simulink model "OuterLoop"  (R2023b)
settings: Solver=VariableStepAuto  StartTime=0.0  StopTime=10.0  RelTol=1e-3
model workspace (MAT data in the model file):
  TorqueSat = 0.0675
values from neighbouring files (symbols this model uses):
  Jb = Js    (= 0.05116)    [Attitude_OuterLoop.m]    (also in SystemVariables.m)
  K = place(A,B,p)    [Attitude_OuterLoop.m]    (also in BLDC_measures.m = 11200)
  Kt = Ke    (= 0.0675)    [Attitude_OuterLoop.m]    (also in BLDC_measures.m; SystemVariables.m)
libraries: simulink_extras x2
settings Model: Creator=Jorge CM  LastModifiedBy=Jorge CM

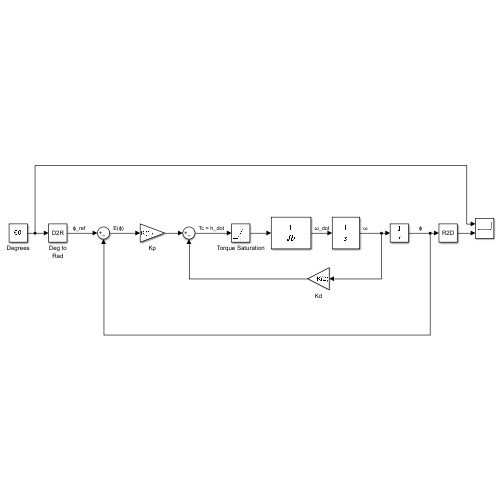
[thumbnail: Simulink's stored preview of the top-level diagram]
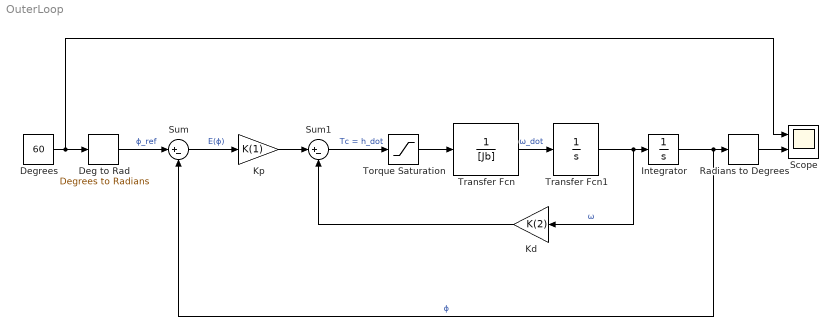
== system OuterLoop ==
  Deg to Rad : simulink_extras/Transformations/Degrees to Radians
  Degrees : Constant  Value=60
  Integrator : Integrator
  Kd : Gain  Gain=K(2)
  Kp : Gain  Gain=K(1)
  Radians to Degrees : simulink_extras/Transformations/Radians to Degrees
  Scope : Scope  NumInputPorts=2
  Sum : Sum  Inputs=|+-
  Sum1 : Sum  Inputs=|+-
  Torque Saturation : Saturate  UpperLimit=Kt  LowerLimit=-Kt
  Transfer Fcn : TransferFcn  Denominator=[Jb]
  Transfer Fcn1 : TransferFcn  Denominator=[1 0]
  wires:
  Degrees/1 -> Scope/1, Deg to Rad/1
  Deg to Rad/1 -> Sum/1  "ϕ_ref"
  Sum/1 -> Kp/1  "E(ϕ)"
  Sum1/1 -> Torque Saturation/1  "Tc = h_dot"
  Transfer Fcn/1 -> Transfer Fcn1/1  "ω_dot"
  Integrator/1 -> Radians to Degrees/1, Sum/2  "ϕ"
  Radians to Degrees/1 -> Scope/2
  Transfer Fcn1/1 -> Kd/1, Integrator/1  "ω"
  Kd/1 -> Sum1/2
  Kp/1 -> Sum1/1
  Torque Saturation/1 -> Transfer Fcn/1
